simulink model "untitled2"  (R2023b)
settings: Solver=FixedStepAuto  StartTime=0.0  StopTime=10.0  RelTol=1e-3
values from neighbouring files (symbols this model uses):
  b1 = b(1,:)    [bicyclekinematicmodel.m]
  b2 = b(2,:)    [bicyclekinematicmodel.m]
undefined symbols (not defined in the file or in its folder): a
libraries: fuzblock x1
settings Model: Creator=samee  LastModifiedBy=samee

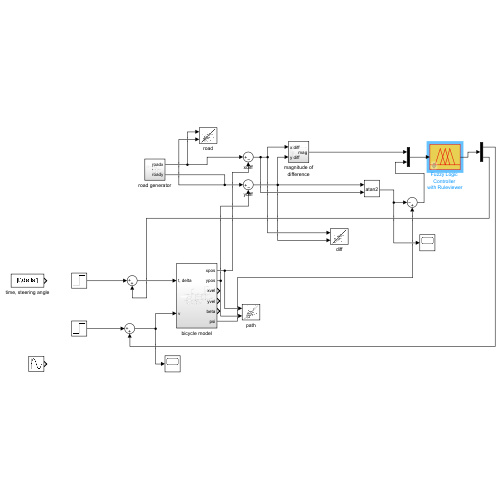
[thumbnail: Simulink's stored preview of the top-level diagram]
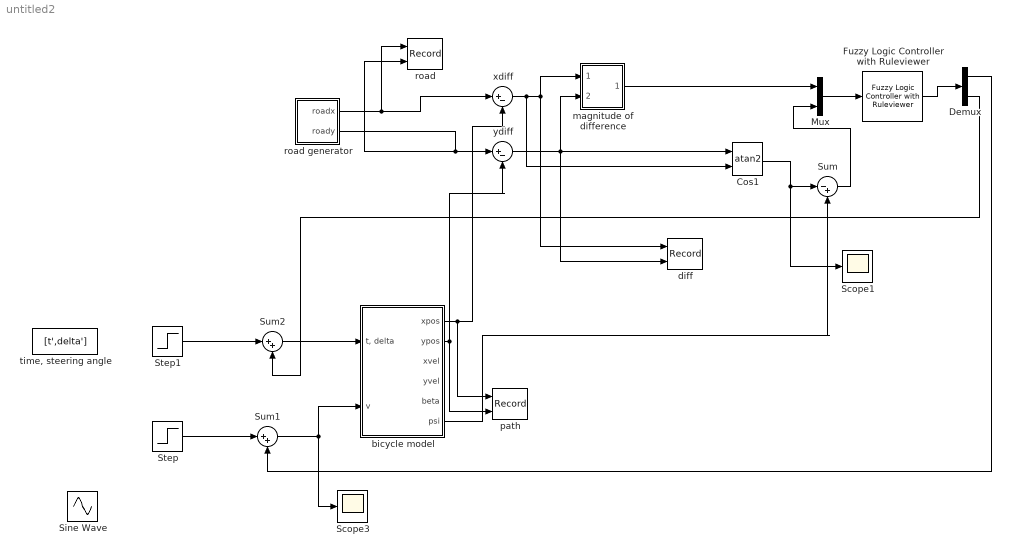
== system untitled2 ==
  Cos1 : Trigonometry  Operator=atan2
  Demux : Demux  Outputs=2
  Fuzzy Logic Controller with Ruleviewer : fuzblock/Fuzzy Logic  Controller  with Ruleviewer  fismatrix=fismatrix  Ts=2
  Mux : Mux  Inputs=2
  Scope1 : Scope
  Scope3 : Scope
  Sine Wave : Sin  Amplitude=30  Frequency=0.125  SampleTime=0
  Step : Step  Time=0.05  SampleTime=0
  Step1 : Step  Time=0.05  SampleTime=0
  Sum : Sum  Inputs=|-+
  Sum1 : Sum  Inputs=|++
  Sum2 : Sum  Inputs=|++
  bicycle model : Subsystem
  diff : Record  FileSettingsInternal="{\"entries\":[{\"content\":{\"excelSettings\":{\"content\":{},\"type\":\"Streamout.ExcelSettings\"}},\"type\":\"Streamout.FileSettingStorage\",\"uuid\":\"\"}],\"packageUris\":[\"http:\\/\\/schema.mathworks.com\\/mf0\\/streamout_blocks\\/R2020a\"],\"version\":\"1.0\"}"  Layout=[1 1]  SignalsInternal="{\"entries\":[{\"content\":{\"signals\":[{\"content\":{\"blockPath\":[],\"dimensions\":[1],\"domain\":\"\",\"lineColor\":\"#7e2f8e\",\"plots\":[1],\"port\":1,\"signalID\":43,\"signalName\":\"xdiff\"},\"type\":\"RecordBlkView.Signal\",\"uuid\":\"\"},{\"content\":{\"blockPath\":[],\"dimensions\":[1],\"domain\":\"\",\"lineColor\":\"#77ac30\",\"plots\":[1],\"port\":2,\"signalID\":46,\"signalName\":\"ydiff\"},\"type\":\"RecordBlkView.Signal\",\"uuid\":\"\"}]},\"type\":\"RecordBlkView.InputSignals\",\"uuid\":\"\"}],\"packageUris\":[\"http:\\/\\/schema.mathworks.com\\/mf0\\/streamout_blocks\\/R2020a\"],\"version\":\"1.0\"}"  VisualizationBindings="{\"xyplotplugin\":{\"info\":[{\"series\":[{\"bindingParametersList\":[{\"parameter\":\"X-Axis\",\"signalID\":43,\"signalName\":\"xdiff\"},{\"parameter\":\"Y-Axis\",\"signalID\":46,\"signalName\":\"ydiff\"}],\"seriesID\":30984}],\"subplotID\":1}]}}"  CompatibilityTag=XY
  magnitude of difference : Subsystem
  path : Record  FileSettingsInternal="{\"entries\":[{\"content\":{\"excelSettings\":{\"content\":{},\"type\":\"Streamout.ExcelSettings\"}},\"type\":\"Streamout.FileSettingStorage\",\"uuid\":\"\"}],\"packageUris\":[\"http:\\/\\/schema.mathworks.com\\/mf0\\/streamout_blocks\\/R2020a\"],\"version\":\"1.0\"}"  Layout=[1 1]  SignalsInternal="{\"entries\":[{\"content\":{\"signals\":[{\"content\":{\"blockPath\":[],\"dimensions\":[1],\"domain\":\"\",\"lineColor\":\"#4dbeee\",\"port\":1,\"signalID\":51,\"signalName\":\"bicycle model:1\"},\"type\":\"RecordBlkView.Signal\",\"uuid\":\"\"},{\"content\":{\"blockPath\":[],\"dimensions\":[1],\"domain\":\"\",\"lineColor\":\"#a2142f\",\"port\":2,\"signalID\":54,\"signalName\":\"bicycle model:2\"},\"type\":\"RecordBlkView.Signal\",\"uuid\":\"\"}]},\"type\":\"RecordBlkView.InputSignals\",\"uuid\":\"\"}],\"packageUris\":[\"http:\\/\\/schema.mathworks.com\\/mf0\\/streamout_blocks\\/R2020a\"],\"version\":\"1.0\"}"  VisualizationBindings="{\"xyplotplugin\":{\"info\":[{\"series\":[],\"subplotID\":1}]}}"  CompatibilityTag=XY
  road : Record  FileSettingsInternal="{\"entries\":[{\"content\":{\"excelSettings\":{\"content\":{},\"type\":\"Streamout.ExcelSettings\"}},\"type\":\"Streamout.FileSettingStorage\",\"uuid\":\"\"}],\"packageUris\":[\"http:\\/\\/schema.mathworks.com\\/mf0\\/streamout_blocks\\/R2020a\"],\"version\":\"1.0\"}"  Layout=[1 1]  SignalsInternal="{\"entries\":[{\"content\":{\"signals\":[{\"content\":{\"blockPath\":[],\"dimensions\":[1],\"domain\":\"\",\"lineColor\":\"#139fff\",\"plots\":[1],\"port\":1,\"signalID\":35,\"signalName\":\"road generator:1\"},\"type\":\"RecordBlkView.Signal\",\"uuid\":\"\"},{\"content\":{\"blockPath\":[],\"dimensions\":[1],\"domain\":\"\",\"lineColor\":\"#ff6929\",\"plots\":[1],\"port\":2,\"signalID\":38,\"signalName\":\"road generator:2\"},\"type\":\"RecordBlkView.Signal\",\"uuid\":\"\"}]},\"type\":\"RecordBlkView.InputSignals\",\"uuid\":\"\"}],\"packageUris\":[\"http:\\/\\/schema.mathworks.com\\/mf0\\/streamout_blocks\\/R2020a\"],\"version\":\"1.0\"}"  VisualizationBindings="{\"xyplotplugin\":{\"info\":[{\"series\":[{\"bindingParametersList\":[{\"parameter\":\"X-Axis\",\"signalID\":35,\"signalName\":\"road generator:1\"},{\"parameter\":\"Y-Axis\",\"signalID\":38,\"signalName\":\"road generator:2\"}],\"seriesID\":100}],\"subplotID\":1}]}}"  CompatibilityTag=XY
  road generator : Subsystem
  "time, steering angle" : FromWorkspace  VariableName=[t',delta']  OutDataTypeStr=double  SampleTime=-1
  xdiff : Sum  Inputs=|+-
  ydiff : Sum  Inputs=|+-
  wires:
  xdiff/1 -> Cos1/2, diff/1, magnitude of difference/1(x diff)
  ydiff/1 -> Cos1/1, diff/2, magnitude of difference/2(y diff)
  bicycle model/1(xpos) -> xdiff/2, path/1
  bicycle model/2(ypos) -> ydiff/2, path/2
  Cos1/1 -> Sum/1, Scope1/1
  Mux/1 -> Fuzzy Logic Controller with Ruleviewer/1
  Fuzzy Logic Controller with Ruleviewer/1 -> Demux/1
  magnitude of difference/1(mag) -> Mux/1
  road generator/1(roadx) -> xdiff/1, road/1
  road generator/2(roady) -> road/2, ydiff/1
  bicycle model/6(psi) -> Sum/2
  Sum/1 -> Mux/2
  Step/1 -> Sum1/1
  Sum1/1 -> bicycle model/2(v), Scope3/1
  Demux/1 -> Sum1/2
  Step1/1 -> Sum2/1
  Sum2/1 -> bicycle model/1("t, delta")
  Demux/2 -> Sum2/2

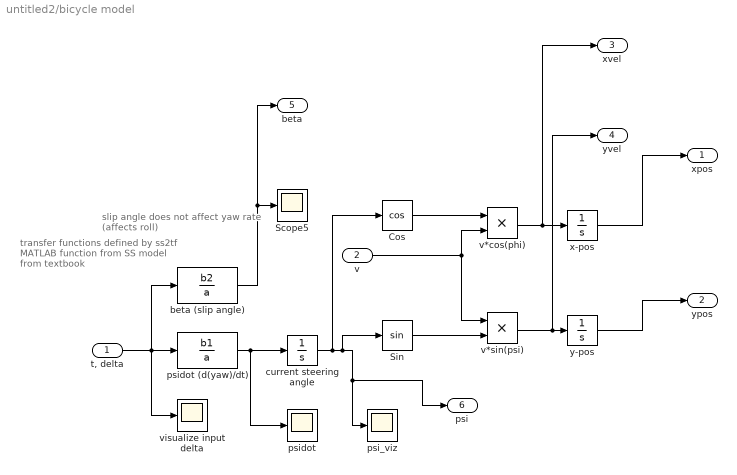
== system untitled2/bicycle model ==
  note: transfer functions defined by ss2tf
      | MATLAB function from SS model
      | from textbook
  note: slip angle does not affect yaw rate
      | (affects roll)
  "t, delta" : Inport
  v : Inport  Port=2
  Cos : Trigonometry  Operator=cos
  Scope5 : Scope
  Sin : Trigonometry
  beta (slip angle) : TransferFcn  Numerator=b2  Denominator=a  ContinuousStateAttributes='beta'
  current steering angle : Integrator
  psi_viz : Scope
  psidot : Scope
  psidot (d(yaw)/dt) : TransferFcn  Numerator=b1  Denominator=a  ContinuousStateAttributes='psidot'
  v*cos(phi) : Product
  v*sin(psi) : Product
  visualize input delta : Scope
  x-pos : Integrator
  y-pos : Integrator
  xpos : Outport
  ypos : Outport  Port=2
  xvel : Outport  Port=3
  yvel : Outport  Port=4
  beta : Outport  Port=5
  psi : Outport  Port=6
  wires:
  psidot (d(yaw)/dt)/1 -> current steering angle/1, psidot/1
  v*sin(psi)/1 -> yvel/1, y-pos/1
  current steering angle/1 -> psi/1, psi_viz/1, Sin/1, Cos/1
  "t, delta"/1 -> visualize input delta/1, beta (slip angle)/1, psidot (d(yaw)/dt)/1
  Sin/1 -> v*sin(psi)/2
  v/1 -> v*sin(psi)/1, v*cos(phi)/2
  v*cos(phi)/1 -> xvel/1, x-pos/1
  beta (slip angle)/1 -> beta/1, Scope5/1
  Cos/1 -> v*cos(phi)/1
  y-pos/1 -> ypos/1
  x-pos/1 -> xpos/1

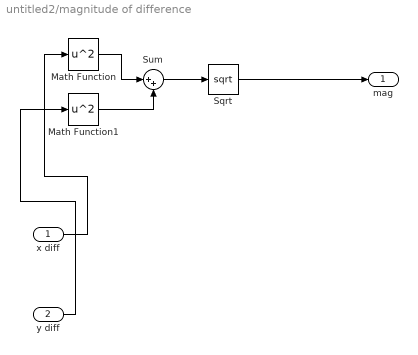
== system untitled2/magnitude of difference ==
  x diff : Inport
  y diff : Inport  Port=2
  Math Function : Math  Operator=square
  Math Function1 : Math  Operator=square
  Sqrt : Sqrt
  Sum : Sum  Inputs=|++
  mag : Outport
  wires:
  Math Function/1 -> Sum/1
  Sum/1 -> Sqrt/1
  Math Function1/1 -> Sum/2
  y diff/1 -> Math Function1/1
  Sqrt/1 -> mag/1
  x diff/1 -> Math Function/1

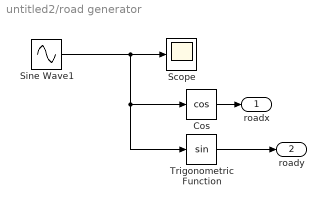
== system untitled2/road generator ==
  Cos : Trigonometry  Operator=cos
  Scope : Scope
  Sine Wave1 : Sin  Frequency=0.25  SampleTime=0
  Trigonometric Function : Trigonometry
  roadx : Outport
  roady : Outport  Port=2
  wires:
  Sine Wave1/1 -> Cos/1, Trigonometric Function/1, Scope/1
  Trigonometric Function/1 -> roady/1
  Cos/1 -> roadx/1
